simulink model "F16_openloop"  (Simulink 6.0)
settings: Solver=ode3  StartTime=0.0  StopTime=10.0  FixedStep=0.02  RelTol=1e-3
values from neighbouring files (symbols this model uses):
  fi_flag_Simulink = 1    [runF16model.m]
  init_dlef = uu(5)    [runF16model.m]
  init_u = uu(1:4)    [runF16model.m]
  init_x = xu(1:14)    [runF16model.m]
libraries: simulink_extras x1
settings Model: Creator=larssonneveldt  LastModifiedBy=larssonneveldt
settings DataIOCC: SignalLoggingName=sigsOut
settings OptimizationCC: ExpressionDepthLimit=2147483647  SimCompilerOptimization=Off
settings DebuggingCC: SaveWithParameterizedLinksMsg=none  SolverPrmCheckMsg=none  MultiTaskDSMMsg=warning  MultiTaskCondExecSysMsg=none  FcnCallInpInsideContextMsg=Use local settings  StateNameClashWarn=warning  StrictBusMsg=None
settings HardwareCC: TargetHWDeviceType=32-bit Generic  TargetUnknown=on  ProdEqTarget=off
settings RTWCC: IncludeERTFirstTime=on  RTWCompilerOptimization=Off
settings CodeAppCC: CustomSymbolStrType=$N$R$M

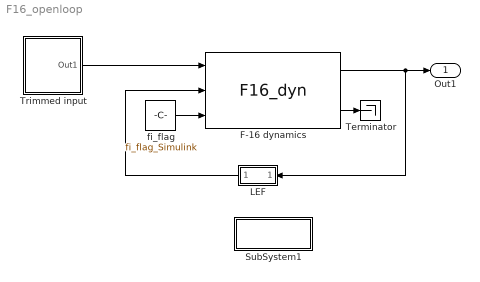
== system F16_openloop ==
  F-16 dynamics : S-Function  FunctionName=F16_dyn  Parameters=init_x
      mask Display: image(imread('aerodata/f16.jpg'))
  LEF : Subsystem  Orientation=left
      mask Display: port_label('output', 1, 'dlef')
  SubSystem1 : Subsystem
      settings: OpenFcn=edit(fullfile(cd,'F16_dyn.c'))
      mask Display: disp('F16_dyn.c');
  Terminator : Terminator
  Trimmed input : Subsystem
      mask Display: image(imread('aerodata\f16cockpit.jpg'))
  fi_flag : Constant  Value=fi_flag_Simulink  OutDataType=sfix(16)  OutScaling=2^0
  Out1 : Outport  OutDataType=sfix(16)  OutScaling=2^0
  wires:
  F-16 dynamics/1 -> Out1/1, LEF/1(state)
  Trimmed input/1(Out1) -> F-16 dynamics/1
  fi_flag/1 -> F-16 dynamics/3
  LEF/1("delta_lef ") -> F-16 dynamics/2
  F-16 dynamics/2 -> Terminator/1

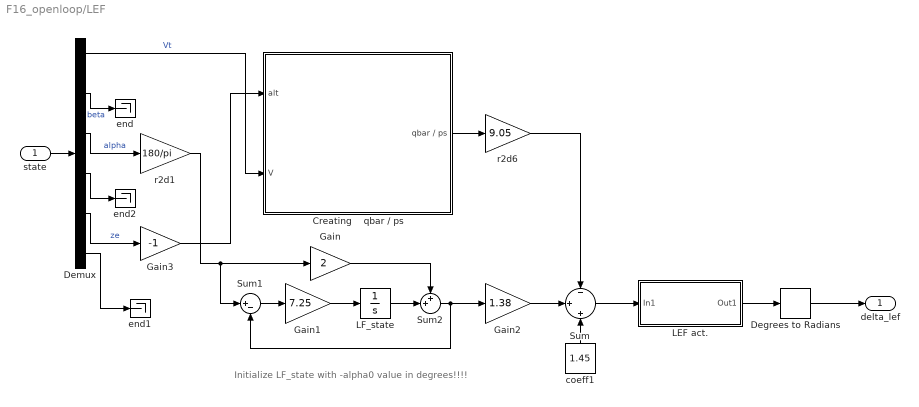
== system F16_openloop/LEF ==
  note: Initialize LF_state with -alpha0 value in degrees!!!!
  state : Inport  OutDataType=sfix(16)  OutScaling=2^0
  Creating    qbar / ps : Subsystem
  Degrees to Radians : simulink_extras/Transformations/Degrees to Radians  SystemSampleTime=-1
  Demux : Demux  Outputs=[1 1 1 9 1 1]
  Gain : Gain  Gain=2  ParameterDataType=sfix(16)  ParameterScaling=2^0  OutDataType=sfix(16)  OutScaling=2^0  SaturateOnIntegerOverflow=on
  Gain1 : Gain  Gain=7.25  ParameterDataType=sfix(16)  ParameterScaling=2^0  OutDataType=sfix(16)  OutScaling=2^0  SaturateOnIntegerOverflow=on
  Gain2 : Gain  Gain=1.38  ParameterDataType=sfix(16)  ParameterScaling=2^0  OutDataType=sfix(16)  OutScaling=2^0  SaturateOnIntegerOverflow=on
  Gain3 : Gain  Gain=-1  ParameterDataType=sfix(16)  ParameterScaling=2^0  OutDataType=sfix(16)  OutScaling=2^0  SaturateOnIntegerOverflow=on
  LEF act. : Subsystem
  LF_state : Integrator  InitialCondition=-init_x(3)*180/pi
  Sum : Sum  Inputs=-|+|+  OutDataType=sfix(16)  OutScaling=2^0  SaturateOnIntegerOverflow=on  InputSameDT=on
  Sum1 : Sum  Inputs=|+-  OutDataType=sfix(16)  OutScaling=2^0  SaturateOnIntegerOverflow=on  InputSameDT=on
  Sum2 : Sum  Inputs=++|  OutDataType=sfix(16)  OutScaling=2^0  SaturateOnIntegerOverflow=on  InputSameDT=on
  coeff1 : Constant  Orientation=up  Value=1.45  OutDataType=sfix(16)  OutScaling=2^0
  end : Terminator
  end1 : Terminator
  end2 : Terminator
  r2d1 : Gain  Gain=180/pi  ParameterDataType=sfix(16)  ParameterScaling=2^0  OutDataType=sfix(16)  OutScaling=2^0  SaturateOnIntegerOverflow=on
  r2d6 : Gain  Gain=9.05  ParameterDataType=sfix(16)  ParameterScaling=2^0  OutDataType=sfix(16)  OutScaling=2^0  SaturateOnIntegerOverflow=on
  "delta_lef " : Outport  OutDataType=sfix(16)  OutScaling=2^0
  wires:
  Degrees to Radians/1 -> "delta_lef "/1
  Gain3/1 -> Creating    qbar / ps/1(alt)
  LEF act./1(Out1) -> Degrees to Radians/1
  Sum/1 -> LEF act./1(In1)
  state/1 -> Demux/1
  Sum1/1 -> Gain1/1
  Gain1/1 -> LF_state/1
  Gain/1 -> Sum2/1
  Gain2/1 -> Sum/2
  coeff1/1 -> Sum/3
  Sum2/1 -> Sum1/2, Gain2/1
  LF_state/1 -> Sum2/2
  r2d1/1 -> Sum1/1, Gain/1
  Creating    qbar / ps/1(qbar / ps) -> r2d6/1
  r2d6/1 -> Sum/1
  Demux/1 -> Creating    qbar / ps/2(V)  "Vt"
  Demux/2 -> end/1  "beta"
  Demux/3 -> r2d1/1  "alpha"
  Demux/4 -> end2/1
  Demux/5 -> Gain3/1  "ze"
  Demux/6 -> end1/1

== system F16_openloop/SubSystem1 ==

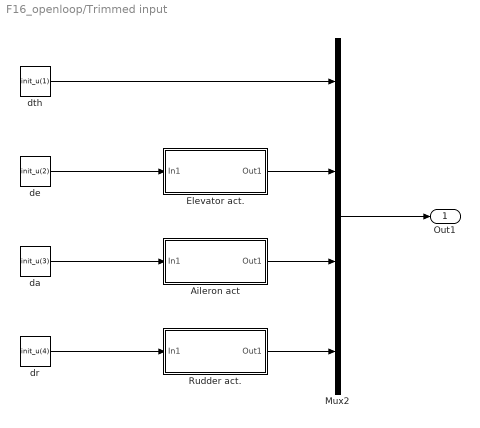
== system F16_openloop/Trimmed input ==
  Aileron act : Subsystem
      mask Display:
      | port_label('output', 1, 'da')
      | port_label('input', 1, 'da_ref')
  Elevator act. : Subsystem
      mask Display:
      | port_label('output', 1, 'de')
      | port_label('input', 1, 'de_ref')
  Mux2 : Mux
  Rudder act. : Subsystem
      mask Display:
      | port_label('output', 1, 'dr')
      | port_label('input', 1, 'dr_ref')
  da : Constant  Value=init_u(3)  OutDataType=sfix(16)  OutScaling=2^0
  de : Constant  Value=init_u(2)  OutDataType=sfix(16)  OutScaling=2^0
  dr : Constant  Value=init_u(4)  OutDataType=sfix(16)  OutScaling=2^0
  dth : Constant  Value=init_u(1)  OutDataType=sfix(16)  OutScaling=2^0
  Out1 : Outport  OutDataType=sfix(16)  OutScaling=2^0
  wires:
  Mux2/1 -> Out1/1
  Elevator act./1(Out1) -> Mux2/2
  Aileron act/1(Out1) -> Mux2/3
  Rudder act./1(Out1) -> Mux2/4
  dth/1 -> Mux2/1
  de/1 -> Elevator act./1(In1)
  da/1 -> Aileron act/1(In1)
  dr/1 -> Rudder act./1(In1)

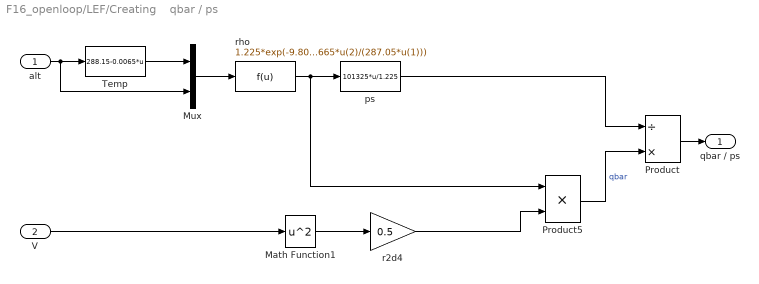
== system F16_openloop/LEF/Creating    qbar / ps ==
  alt : Inport  OutDataType=sfix(16)  OutScaling=2^0
  V : Inport  Port=2  OutDataType=sfix(16)  OutScaling=2^0
  Math Function1 : Math  Operator=square  OutDataType=sfix(16)  OutScaling=2^0  SaturateOnIntegerOverflow=on
  Mux : Mux  Inputs=2
  Product : Product  Inputs=/*  OutDataType=sfix(16)  OutScaling=2^0  SaturateOnIntegerOverflow=on  InputSameDT=on
  Product5 : Product  Inputs=**  OutDataType=sfix(16)  OutScaling=2^0  SaturateOnIntegerOverflow=on  InputSameDT=on
  Temp : Fcn  Expr=288.15-0.0065*u
  ps : Fcn  Expr=101325*u/1.225
  r2d4 : Gain  Gain=0.5  ParameterDataType=sfix(16)  ParameterScaling=2^0  OutDataType=sfix(16)  OutScaling=2^0  SaturateOnIntegerOverflow=on
  rho : Fcn  Expr=1.225*exp(-9.80665*u(2)/(287.05*u(1)))
  qbar / ps : Outport  OutDataType=sfix(16)  OutScaling=2^0
  wires:
  ps/1 -> Product/1
  rho/1 -> Product5/1, ps/1
  Mux/1 -> rho/1
  Temp/1 -> Mux/1
  alt/1 -> Mux/2, Temp/1
  Math Function1/1 -> r2d4/1
  r2d4/1 -> Product5/2
  Product5/1 -> Product/2  "qbar"
  Product/1 -> qbar / ps/1
  V/1 -> Math Function1/1

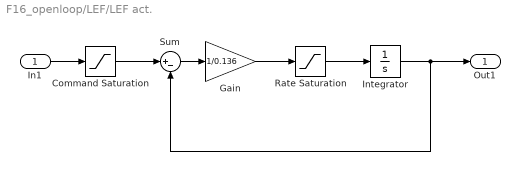
== system F16_openloop/LEF/LEF act. ==
  In1 : Inport  OutDataType=sfix(16)  OutScaling=2^0
  Command Saturation : Saturate  UpperLimit=25  LowerLimit=0
  Gain : Gain  Gain=1/0.136  ParameterDataType=sfix(16)  ParameterScaling=2^0  OutDataType=sfix(16)  OutScaling=2^0  SaturateOnIntegerOverflow=on
  "Integrator " : Integrator  InitialCondition=init_dlef*180/pi  UpperSaturationLimit=25  LowerSaturationLimit=-25
  Rate Saturation : Saturate  UpperLimit=25  LowerLimit=-25
  Sum : Sum  Inputs=|+-  OutDataType=sfix(16)  OutScaling=2^0  SaturateOnIntegerOverflow=on  InputSameDT=on
  Out1 : Outport  OutDataType=sfix(16)  OutScaling=2^0
  wires:
  "Integrator "/1 -> Sum/2, Out1/1
  Rate Saturation/1 -> "Integrator "/1
  Gain/1 -> Rate Saturation/1
  Sum/1 -> Gain/1
  Command Saturation/1 -> Sum/1
  In1/1 -> Command Saturation/1

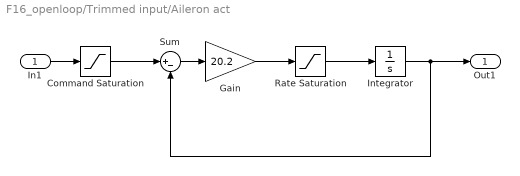
== system F16_openloop/Trimmed input/Aileron act ==
  In1 : Inport  OutDataType=sfix(16)  OutScaling=2^0
  Command Saturation : Saturate  UpperLimit=21.5*pi/180  LowerLimit=-21.5*pi/180
  Gain : Gain  Gain=20.2  ParameterDataType=sfix(16)  ParameterScaling=2^0  OutDataType=sfix(16)  OutScaling=2^0  SaturateOnIntegerOverflow=on
  "Integrator " : Integrator  InitialCondition=init_u(3)  UpperSaturationLimit=21.5  LowerSaturationLimit=-21.5
  Rate Saturation : Saturate  UpperLimit=80*pi/180  LowerLimit=-80*pi/180
  Sum : Sum  Inputs=|+-  OutDataType=sfix(16)  OutScaling=2^0  SaturateOnIntegerOverflow=on  InputSameDT=on
  Out1 : Outport  OutDataType=sfix(16)  OutScaling=2^0
  wires:
  "Integrator "/1 -> Sum/2, Out1/1
  Rate Saturation/1 -> "Integrator "/1
  Gain/1 -> Rate Saturation/1
  Sum/1 -> Gain/1
  Command Saturation/1 -> Sum/1
  In1/1 -> Command Saturation/1

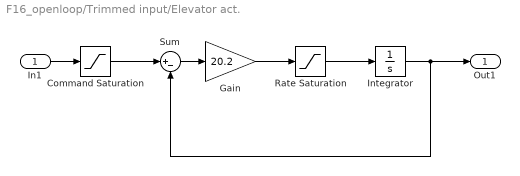
== system F16_openloop/Trimmed input/Elevator act. ==
  In1 : Inport  OutDataType=sfix(16)  OutScaling=2^0
  Command Saturation : Saturate  UpperLimit=25*pi/180  LowerLimit=-25*pi/180
  Gain : Gain  Gain=20.2  ParameterDataType=sfix(16)  ParameterScaling=2^0  OutDataType=sfix(16)  OutScaling=2^0  SaturateOnIntegerOverflow=on
  "Integrator " : Integrator  InitialCondition=init_u(2)  UpperSaturationLimit=25  LowerSaturationLimit=-25
  Rate Saturation : Saturate  UpperLimit=60*pi/180  LowerLimit=-60*pi/180
  Sum : Sum  Inputs=|+-  OutDataType=sfix(16)  OutScaling=2^0  SaturateOnIntegerOverflow=on  InputSameDT=on
  Out1 : Outport  OutDataType=sfix(16)  OutScaling=2^0
  wires:
  "Integrator "/1 -> Sum/2, Out1/1
  Rate Saturation/1 -> "Integrator "/1
  Gain/1 -> Rate Saturation/1
  Sum/1 -> Gain/1
  Command Saturation/1 -> Sum/1
  In1/1 -> Command Saturation/1

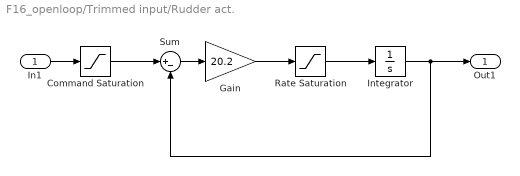
== system F16_openloop/Trimmed input/Rudder act. ==
  In1 : Inport  OutDataType=sfix(16)  OutScaling=2^0
  Command Saturation : Saturate  UpperLimit=30*pi/180  LowerLimit=-30*pi/180
  Gain : Gain  Gain=20.2  ParameterDataType=sfix(16)  ParameterScaling=2^0  OutDataType=sfix(16)  OutScaling=2^0  SaturateOnIntegerOverflow=on
  "Integrator " : Integrator  InitialCondition=init_u(4)  UpperSaturationLimit=25  LowerSaturationLimit=-25
  Rate Saturation : Saturate  UpperLimit=120*pi/180  LowerLimit=-120*pi/180
  Sum : Sum  Inputs=|+-  OutDataType=sfix(16)  OutScaling=2^0  SaturateOnIntegerOverflow=on  InputSameDT=on
  Out1 : Outport  OutDataType=sfix(16)  OutScaling=2^0
  wires:
  In1/1 -> Command Saturation/1
  Command Saturation/1 -> Sum/1
  Sum/1 -> Gain/1
  Gain/1 -> Rate Saturation/1
  Rate Saturation/1 -> "Integrator "/1
  "Integrator "/1 -> Out1/1, Sum/2
